simulink model "P25_Simulink_Ex2_6"  (R2017a)
settings: Solver=VariableStepAuto  StartTime=0.0  StopTime=50  RelTol=1e-6
settings Model: Creator=phylab  LastModifiedBy=phylab

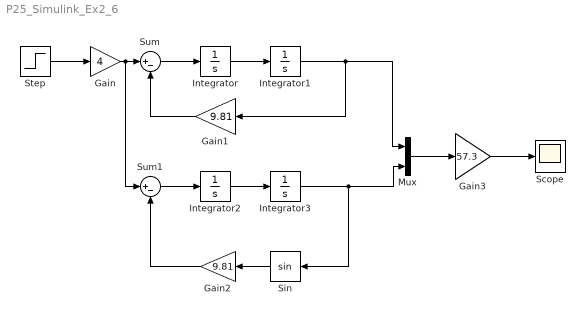
== system P25_Simulink_Ex2_6 ==
  Gain : Gain  Gain=4
  Gain1 : Gain  Gain=9.81
  Gain2 : Gain  Gain=9.81
  Gain3 : Gain  Gain=57.3
  Integrator{,1..3} (4 alike) : Integrator
  Mux : Mux  Inputs=2
  Scope : Scope
  Sin : Trigonometry
  Step : Step  SampleTime=0
  Sum : Sum  Inputs=|+-
  Sum1 : Sum  Inputs=|+-
  wires:
  Step/1 -> Gain/1
  Gain/1 -> Sum1/1, Sum/1
  Sum/1 -> Integrator/1
  Integrator/1 -> Integrator1/1
  Integrator1/1 -> Gain1/1, Mux/1
  Gain1/1 -> Sum/2
  Sum1/1 -> Integrator2/1
  Integrator2/1 -> Integrator3/1
  Integrator3/1 -> Sin/1, Mux/2
  Gain2/1 -> Sum1/2
  Sin/1 -> Gain2/1
  Mux/1 -> Gain3/1
  Gain3/1 -> Scope/1
